simulink model "SCRReferenceApplication"  (R2024a)
settings: Solver=ode23tb  StartTime=0.0  StopTime=inf  RelTol=2e-1
model workspace (MAT data in the model file):
  EngPwr = 352122.842504
  EngWc = 4.047
  Tdiff = 849
  Tlim = 1000
  VEH : object (value not decoded)
libraries: simulink x7, vehdynlibtirecommon x4, autolibutils x4, sim3dlib x3, sharedtransform x2, vehdynlibtire x1, sim3dautolib x1, vehdynlibsteering x1, dspnetwork x1, autolibshared x1
(part 2 of 2)

== matlab function SCRReferenceApplication/MATLAB Function ==
  data: u input; steer output double
function steer = parse_steer(u)
%#codegen
% Parse steering value sent as ASCII text, e.g. "25" or "-40"

steer = double(0);

% Count valid bytes (nonzero)
n = 0;
for i = 1:length(u)
    if u(i) ~= 0
        n = n + 1;
    end
end

if n == 0
    return;
end

% Build character buffer
buf = char(zeros(1, n));
k = 1;
for i = 1:length(u)
    if u(i) ~= 0
        buf(k) = char(u(i));
        k = k + 1;
    end
end

% Convert ASCII text to numeric value
v = str2double(buf);

% Keep only valid real scalar
if ~isnan(v) && isreal(v)
    steer = double(v);
else
    steer = double(0);
end
